simulink model "modelWachadla"  (R2017a)
settings: Solver=VariableStepAuto  StartTime=0.0  StopTime=20  MinStep=0.01  RelTol=1e-3  EnableMultiTasking=on
undefined symbols (not defined in the file or in its folder): A0, A120, A150, A180, A30, A60, A90, B0, B120, B150, B180, B30, B60, B90
libraries: fuzblock x1
settings Model: Creator=student  LastModifiedBy=Szwank
settings DataIOCC: SaveFormat=StructureWithTime
settings OptimizationCC: LifeSpan=inf
settings DebuggingCC: SFUnexpectedBacktrackingDiag=warning  SFNoUnconditionalDefaultTransitionDiag=warning  SFExecutionAtInitializationDiag=none
settings HardwareCC: ProdBitPerSizeT=32  ProdBitPerPtrDiffT=32  ProdWordSize=32  ProdHWDeviceType=Specified
settings GRTTargetCC: TargetLangStandard=C89/C90 (ANSI)  GeneratePreprocessorConditionals=Disable all
settings ConfigComp: CovMetricSettings=dw  CovHtmlReporting=on  CovSaveCumulativeToWorkspaceVar=on  CovSaveSingleToWorkspaceVar=on  CovExternalEMLEnable=off

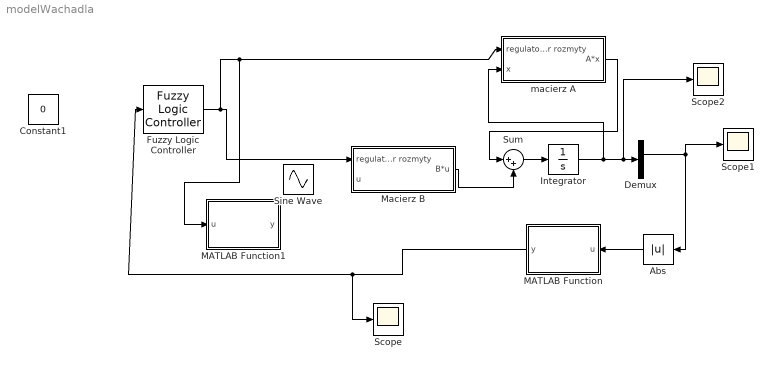
== system modelWachadla ==
  Abs : Abs
  Constant1 : Constant  Value=0
  Demux : Demux
  Fuzzy Logic Controller : fuzblock/Fuzzy Logic  Controller  fis=['modelRozmyty.fis']
  Integrator : Integrator  InitialCondition=[0 pi 0 0.1]
  MATLAB Function : MATLAB Function  TreatAsAtomicUnit=on
  MATLAB Function1 : MATLAB Function  TreatAsAtomicUnit=on
  Macierz B : Subsystem
  Scope : Scope
  Scope1 : Scope
  Scope2 : Scope
  Sine Wave : Sin  Amplitude=0.1  Frequency=0.1  SampleTime=0
  Sum : Sum  Inputs=|++
  "macierz A " : Subsystem
  wires:
  Fuzzy Logic Controller/1 -> MATLAB Function1/1(u), "macierz A "/1(regulator rozmyty), Macierz B/1("regulator rozmyty ")
  Sum/1 -> Integrator/1
  Demux/2 -> Abs/1, Scope1/1
  Abs/1 -> MATLAB Function/1(u)
  MATLAB Function/1(y) -> Scope/1, Fuzzy Logic Controller/1
  "macierz A "/1(A*x) -> Sum/1
  Macierz B/1(B*u) -> Sum/2
  Integrator/1 -> Scope2/1, Demux/1, "macierz A "/2("x ")

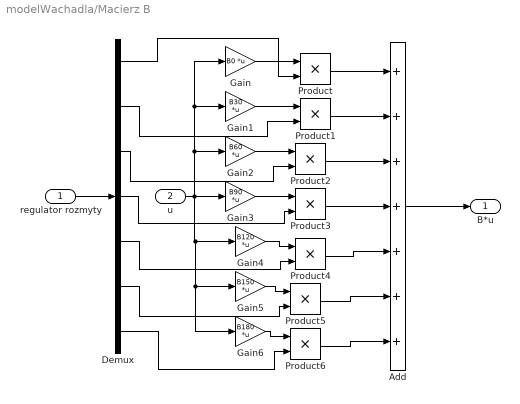
== system modelWachadla/Macierz B ==
  "regulator rozmyty " : Inport
  "u " : Inport  Port=2
  Add : Sum  Inputs=+++++++
  Demux : Demux  Outputs=7
  Gain : Gain  Gain=B0  Multiplication=Matrix(K*u)
  Gain1 : Gain  Gain=B30  Multiplication=Matrix(K*u)
  Gain2 : Gain  Gain=B60  Multiplication=Matrix(K*u)
  Gain3 : Gain  Gain=B90  Multiplication=Matrix(K*u)
  Gain4 : Gain  Gain=B120  Multiplication=Matrix(K*u)
  Gain5 : Gain  Gain=B150  Multiplication=Matrix(K*u)
  Gain6 : Gain  Gain=B180  Multiplication=Matrix(K*u)
  Product{,1..6} (7 alike) : Product
  B*u : Outport
  wires:
  "regulator rozmyty "/1 -> Demux/1
  Add/1 -> B*u/1
  Demux/1 -> Product/2
  "u "/1 -> Gain6/1, Gain5/1, Gain4/1, Gain2/1, Gain1/1, Gain/1, Gain3/1
  Gain/1 -> Product/1
  Gain1/1 -> Product1/1
  Demux/7 -> Product6/2
  Gain6/1 -> Product6/1
  Gain5/1 -> Product5/1
  Gain4/1 -> Product4/1
  Gain3/1 -> Product3/1
  Gain2/1 -> Product2/1
  Demux/2 -> Product1/2
  Demux/3 -> Product2/2
  Demux/4 -> Product3/2
  Demux/5 -> Product4/2
  Demux/6 -> Product5/2
  Product/1 -> Add/1
  Product1/1 -> Add/2
  Product2/1 -> Add/3
  Product3/1 -> Add/4
  Product4/1 -> Add/5
  Product5/1 -> Add/6
  Product6/1 -> Add/7

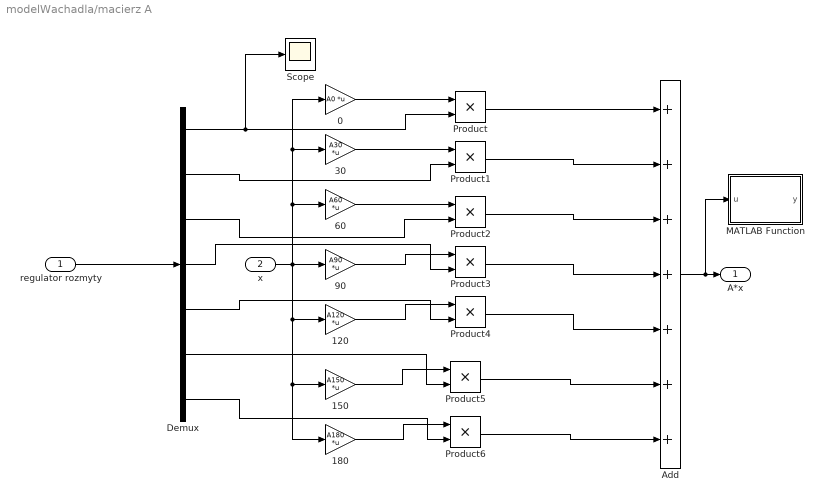
== system modelWachadla/macierz A  ==
  regulator rozmyty : Inport
  "x " : Inport  Port=2
  0 : Gain  Gain=A0  Multiplication=Matrix(K*u)
  120 : Gain  Gain=A120  Multiplication=Matrix(K*u)
  150 : Gain  Gain=A150  Multiplication=Matrix(K*u)
  180 : Gain  Gain=A180  Multiplication=Matrix(K*u)
  "30 " : Gain  Gain=A30  Multiplication=Matrix(K*u)
  60 : Gain  Gain=A60  Multiplication=Matrix(K*u)
  90 : Gain  Gain=A90  Multiplication=Matrix(K*u)
  Add : Sum  Inputs=+++++++
  Demux : Demux  Outputs=7
  MATLAB Function : MATLAB Function  TreatAsAtomicUnit=on
  Product{,1..6} (7 alike) : Product
  Scope : Scope
  A*x : Outport
  wires:
  regulator rozmyty/1 -> Demux/1
  Add/1 -> MATLAB Function/1(u), A*x/1
  "x "/1 -> 120/1, 150/1, 180/1, 0/1, "30 "/1, 60/1, 90/1
  0/1 -> Product/1
  Demux/1 -> Scope/1, Product/2
  "30 "/1 -> Product1/1
  60/1 -> Product2/1
  90/1 -> Product3/1
  120/1 -> Product4/1
  150/1 -> Product5/1
  180/1 -> Product6/1
  Demux/7 -> Product6/2
  Demux/6 -> Product5/2
  Demux/5 -> Product4/2
  Demux/4 -> Product3/2
  Demux/3 -> Product2/2
  Demux/2 -> Product1/2
  Product/1 -> Add/1
  Product1/1 -> Add/2
  Product2/1 -> Add/3
  Product3/1 -> Add/4
  Product4/1 -> Add/5
  Product5/1 -> Add/6
  Product6/1 -> Add/7

== matlab function modelWachadla/MATLAB Function1 ==
  data: u input; y output
function y = fcn(u)
%% Linearyzacja w punktach pracy
[A30,B30] = linearyzacja(pi/6);
[A60,B60] = linearyzacja(pi/3);
[A90,B90] = linearyzacja(pi/2);
[A120,B120] = linearyzacja(pi*4/6);
[A150,B150] = linearyzacja(pi*5/6);
[A180,B180] = linearyzacja(pi-0.001);

[A0,B0]=linearyzacja(0.00000000000000000000000000001);
A0(3:4,2)=[125.66;111.52];%%UWAGA LINEARYZACJA JEST ZLE WYKONANA DLA ALFA RÓWNEGO 0 UWAGA%%
A90(3,2)=0;
A90(4,3)=0;
A180(3:4,2)=[0;0];
B90(4)=0;
     

y = u(1)*A0+u(2)*A30+u(3)*A60+u(4)*A90+u(5)*A120+u(6)*A150+u(7)*A180;

== matlab function modelWachadla/MATLAB Function ==
  data: u input; y output
function y = fcn(u)

g=u*180/pi;
if(g>180)
    reszta=rem(g,180);
    if(rem(fix(g/180),2)==1)
        g=180-reszta;
    else
        g=reszta;
    end

end
y = g;

== matlab function modelWachadla/macierz A /MATLAB Function ==
  data: u input; y output
function y = fcn(u)

y = u;
